simulink model "krause_model_bodine"  (R2017a)
settings: Solver=FixedStepAuto  StartTime=0.0  StopTime=0.4  FixedStep=1e-5  RelTol=1e-3
values from neighbouring files (symbols this model uses):
  B = 0.000124    [krause_model_params.m]
  J = 0.001    [krause_model_params.m]
  Llr = 0.0518    [krause_model_params.m]
  Lls = 0.0222    [krause_model_params.m]
  Lmlstar = 1/(1/Lls+1/Lm+1/Llr)    (= 0.0147655913289)    [krause_model_params.m]
  P = 4    [krause_model_params.m]
  Rr = 12.76    [krause_model_params.m]
  Rs = 14.6    [krause_model_params.m]
libraries: powerlib x12, simulink x1
settings Model: Creator=mircea  LastModifiedBy=mircea

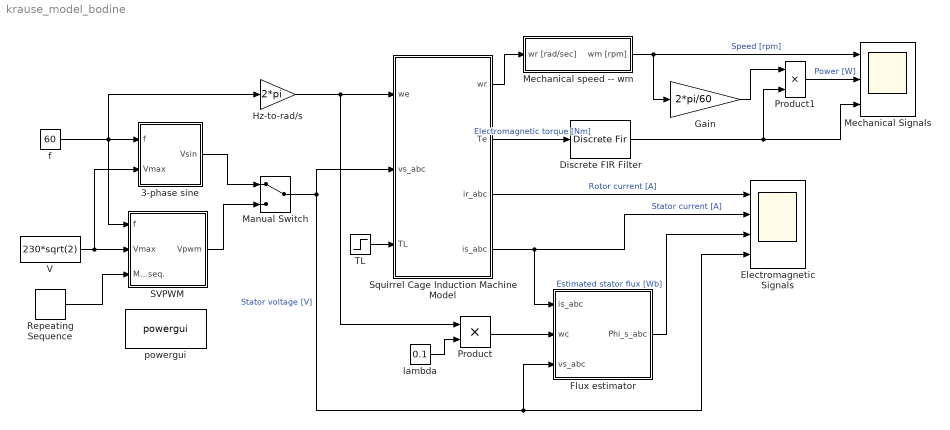
== system krause_model_bodine ==
  3-phase sine : Subsystem
  Discrete FIR Filter : DiscreteFir  Coefficients=ones(1,500)/500
  Electromagnetic Signals : Scope  NumInputPorts=4
  Flux estimator : Subsystem
  Gain : Gain  Gain=2*pi/60
  Hz-to-rad/s : Gain  Gain=2*pi
  Manual Switch : ManualSwitch
  Mechanical Signals : Scope  NumInputPorts=3
  "Mechanical speed -- wm" : Subsystem
  Product : Product
  Product1 : Product
  Repeating Sequence : simulink/Sources/Repeating Sequence  rep_seq_t=[0 0.25 0.5 0.75 1]/(10e3)  rep_seq_y=[1 0 -1 0 1]
  SVPWM : Subsystem
  Squirrel Cage Induction Machine Model : Subsystem
  TL : Step  Time=0.2  After=0.7602
  V : Constant  Value=230*sqrt(2)
  f : Constant  Value=60
  lambda : Constant  Value=0.1
  powergui : powerlib/powergui  Priority=1  SimulationMode=Discrete  SampleTime=1e-5  frequency=60  Iterations=50  frequencyindice=0  Pbase=100e6  ErrMax=1e-4  UnitsV=kV  UnitsW=MW  buscounter=0  FunctionMessages=off  echomessages=off  EnableUseOfTLC=off  CurrentSourceSwitches=off  DisableSnubberDevices=off  DisableRonSwitches=off  DisableVfSwitches=off  DisplayEquations=off  SolverType=Tustin/Backward Euler (TBE)  Interpol=off  ExternalGateDelay=off  methode=off  Ts=100  x0status=blocks  SPID=off  SwTol=0  HookPort=off  RestoreLinks=warning  ResistiveCurrentMeasurement=off  Frange=[0:2:500]  Ylog=off  Xlog=on  ShowGrid=off  save=off  variable=ZData  structure=0  ZoomFFT=off  StartTime=0.0  cycles=1  DisplayStyle=1  fundamental=60  FreqAxis=off  MaxFrequency=1000  frequencyindicesteady=1  RmsSteady=1  display=off
  wires:
  TL/1 -> Squirrel Cage Induction Machine Model/3(TL)
  Squirrel Cage Induction Machine Model/4(is_abc) -> Electromagnetic Signals/2, Flux estimator/1(is_abc)  "Stator current [A]"
  Squirrel Cage Induction Machine Model/3(ir_abc) -> Electromagnetic Signals/1  "Rotor current [A]"
  Product/1 -> Flux estimator/2(wc)
  Flux estimator/1(Phi_s_abc) -> Electromagnetic Signals/3  "Estimated stator flux [Wb]"
  f/1 -> 3-phase sine/1(f), SVPWM/1(f), Hz-to-rad/s/1
  lambda/1 -> Product/2
  Squirrel Cage Induction Machine Model/1(wr) -> "Mechanical speed -- wm"/1(wr [rad/sec])
  "Mechanical speed -- wm"/1(wm [rpm]) -> Mechanical Signals/1, Gain/1  "Speed [rpm]"
  V/1 -> 3-phase sine/2(Vmax), SVPWM/2(Vmax)
  Squirrel Cage Induction Machine Model/2(Te) -> Discrete FIR Filter/1  "Electromagnetic torque [Nm]"
  Product1/1 -> Mechanical Signals/2  "Power [W]"
  Gain/1 -> Product1/1
  Repeating Sequence/1 -> SVPWM/3(Mod. seq.)
  Hz-to-rad/s/1 -> Squirrel Cage Induction Machine Model/1(we), Product/1
  3-phase sine/1(Vsin) -> Manual Switch/1
  SVPWM/1(Vpwm) -> Manual Switch/2
  Manual Switch/1 -> Electromagnetic Signals/4, Flux estimator/3(vs_abc), Squirrel Cage Induction Machine Model/2(vs_abc)  "Stator voltage [V]"
  Discrete FIR Filter/1 -> Mechanical Signals/3, Product1/2

== system krause_model_bodine/3-phase sine ==
  f : Inport
  Vmax : Inport  Port=2
  Clock : Clock
  Constant4 : Constant  Value=2*pi/3*[ 0,-1,1 ]
  Hz-to-rad/s : Gain  Gain=2*pi  SaturateOnIntegerOverflow=on  OutDataTypeStr=Inherit: Same as input  ParamDataTypeStr=Inherit: Same as input
  Product : Product
  Product1 : Product  SaturateOnIntegerOverflow=on  InputSameDT=on  OutDataTypeStr=Inherit: Same as first input
  Sum1 : Sum  SaturateOnIntegerOverflow=on  InputSameDT=on  OutDataTypeStr=Inherit: Same as first input
  Trigonometric Function1 : Trigonometry
  Vsin : Outport
  wires:
  Constant4/1 -> Sum1/2
  Sum1/1 -> Trigonometric Function1/1
  Product1/1 -> Sum1/1
  Hz-to-rad/s/1 -> Product1/2
  Clock/1 -> Product1/1
  Trigonometric Function1/1 -> Product/2
  Vmax/1 -> Product/1
  Product/1 -> Vsin/1
  f/1 -> Hz-to-rad/s/1

== system krause_model_bodine/Flux estimator ==
  is_abc : Inport
  wc : Inport  Port=2
  vs_abc : Inport  Port=3
  Gain1 : Gain  Gain=Rs  SaturateOnIntegerOverflow=on  OutDataTypeStr=Inherit: Same as input  ParamDataTypeStr=Inherit: Same as input
  Integrator : Integrator
  Product : Product
  Subtract : Sum  Inputs=+-
  Sum : Sum  Inputs=|+-
  Phi_s_abc : Outport
  wires:
  Gain1/1 -> Subtract/2
  vs_abc/1 -> Subtract/1
  is_abc/1 -> Gain1/1
  Subtract/1 -> Sum/1
  Sum/1 -> Integrator/1
  Product/1 -> Sum/2
  wc/1 -> Product/2
  Integrator/1 -> Phi_s_abc/1, Product/1

== system krause_model_bodine/Mechanical speed -- wm ==
  wr [rad/sec] : Inport
  Gain : Gain  Gain=2/P
  Gain2 : Gain  Gain=30/pi
  wm [rpm] : Outport
  wires:
  Gain2/1 -> wm [rpm]/1  "wr rpm"
  wr [rad/sec]/1 -> Gain/1
  Gain/1 -> Gain2/1

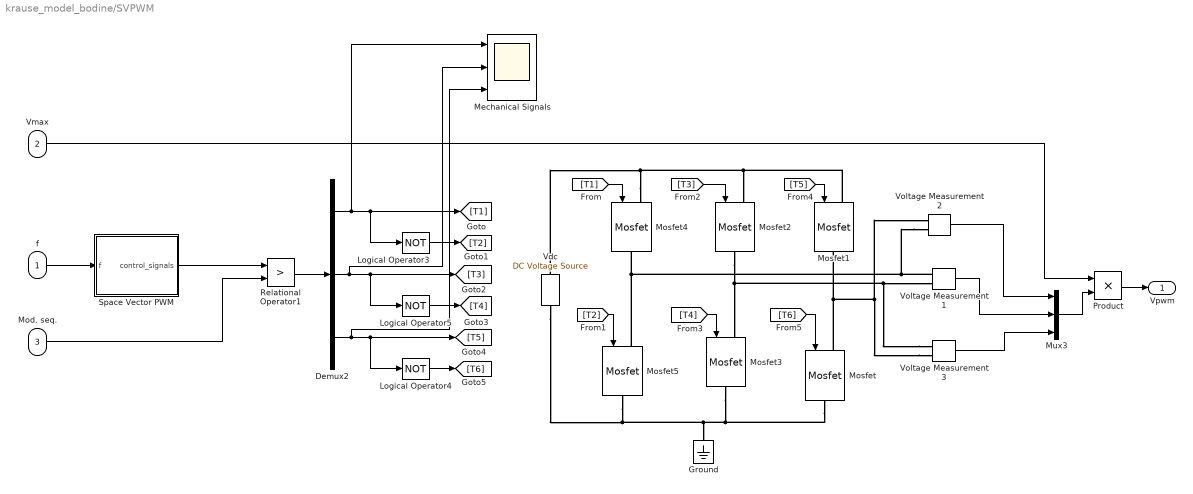
== system krause_model_bodine/SVPWM ==
  f : Inport
  Vmax : Inport  Port=2
  Mod. seq. : Inport  Port=3
  Demux2 : Demux  Outputs=3
  Ground : powerlib/Elements/Ground  LConnTagsString=a
  Logical Operator3 : Logic  Operator=NOT  AllPortsSameDT=off  OutDataTypeStr=boolean
  Logical Operator4 : Logic  Operator=NOT  AllPortsSameDT=off  OutDataTypeStr=boolean
  Logical Operator5 : Logic  Operator=NOT  AllPortsSameDT=off  OutDataTypeStr=boolean
  Mechanical Signals : Scope  NumInputPorts=3
  Mosfet{,1..5} (6 alike) : powerlib/Power Electronics/Mosfet  Ron=0.1  Lon=0  Rd=0.01  Vfd=0  IC=0  Rs=1e5  Cs=inf  Measurements=off
  Mux3 : Mux  Inputs=3
  Product : Product
  Relational Operator1 : RelationalOperator  Operator=>  RndMeth=Nearest
  Space Vector PWM : Subsystem
  Vdc : powerlib/Electrical Sources/DC Voltage Source  Amplitude=1  Measurements=None
  Voltage Measurement1 : powerlib/Measurements/Voltage Measurement  PhasorSimulation=off  OutputType=Complex  PSBequivalent=0
  Voltage Measurement2 : powerlib/Measurements/Voltage Measurement  PhasorSimulation=off  OutputType=Complex  PSBequivalent=0
  Voltage Measurement3 : powerlib/Measurements/Voltage Measurement  PhasorSimulation=off  OutputType=Complex  PSBequivalent=0
  Vpwm : Outport
  wires:
  [T6] -> Mosfet/1
  [T5] -> Mosfet1/1
  [T4] -> Mosfet3/1
  [T3] -> Mosfet2/1
  [T2] -> Mosfet5/1
  [T1] -> Mosfet4/1
  f/1 -> Space Vector PWM/1(f)
  Demux2/3 -> Mechanical Signals/3, [T5], Logical Operator4/1
  Demux2/2 -> Mechanical Signals/2, [T3], Logical Operator5/1
  Logical Operator5/1 -> [T4]
  Demux2/1 -> Mechanical Signals/1, [T1], Logical Operator3/1
  Space Vector PWM/1(control_signals) -> Relational Operator1/1
  Logical Operator4/1 -> [T6]
  Logical Operator3/1 -> [T2]
  Relational Operator1/1 -> Demux2/1
  Mod. seq./1 -> Relational Operator1/2
  Voltage Measurement2/1 -> Mux3/1
  Voltage Measurement1/1 -> Mux3/2
  Voltage Measurement3/1 -> Mux3/3
  Mux3/1 -> Product/2
  Vmax/1 -> Product/1
  Product/1 -> Vpwm/1
  connections:
  Voltage Measurement3/LConn2 -- Mosfet/LConn1 -- Mosfet1/RConn1 -- Voltage Measurement2/LConn1
  Mosfet4/LConn1 -- Mosfet1/LConn1 -- Mosfet2/LConn1 -- Vdc/RConn1
  Voltage Measurement3/LConn1 -- Mosfet3/LConn1 -- Mosfet2/RConn1 -- Voltage Measurement1/LConn2
  Mosfet5/RConn1 -- Mosfet/RConn1 -- Mosfet3/RConn1 -- Ground/LConn1 -- Vdc/LConn1
  Voltage Measurement2/LConn2 -- Voltage Measurement1/LConn1 -- Mosfet4/RConn1 -- Mosfet5/LConn1

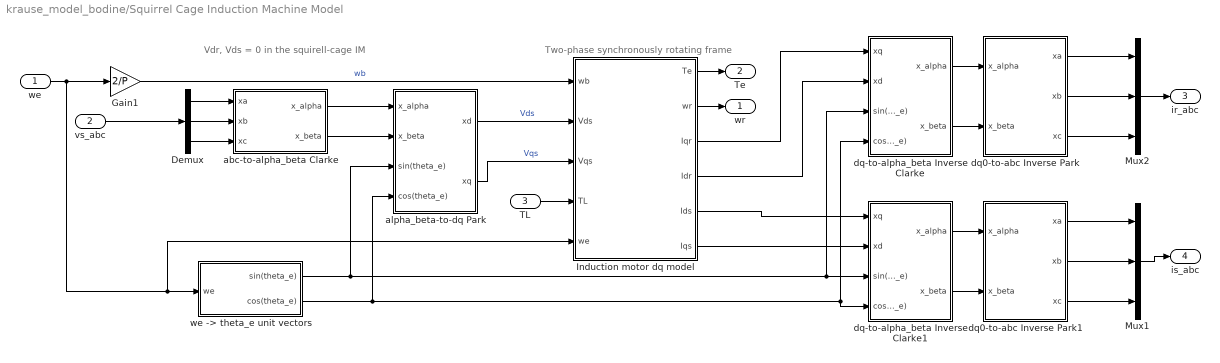
== system krause_model_bodine/Squirrel Cage Induction Machine Model ==
  note: Vdr, Vds = 0 in the squirell-cage IM
  note: Two-phase synchronously rotating frame
  we : Inport
  vs_abc : Inport  Port=2
  TL : Inport  Port=3
  Demux : Demux  Outputs=3
  Gain1 : Gain  Gain=2/P
  Induction motor dq model : Subsystem
  Mux1 : Mux  Inputs=3
  Mux2 : Mux  Inputs=3
  abc-to-alpha_beta Clarke : Subsystem
  alpha_beta-to-dq Park : Subsystem
  dq-to-alpha_beta Inverse Clarke : Subsystem
  dq-to-alpha_beta Inverse Clarke1 : Subsystem
  dq0-to-abc Inverse Park : Subsystem
  dq0-to-abc Inverse Park1 : Subsystem
  "we -> theta_e unit vectors" : Subsystem
  wr : Outport
  Te : Outport  Port=2
  ir_abc : Outport  Port=3
  is_abc : Outport  Port=4
  wires:
  Induction motor dq model/5(Ids) -> dq-to-alpha_beta Inverse Clarke1/1(xq)
  we/1 -> "we -> theta_e unit vectors"/1(we), Induction motor dq model/5(we), Gain1/1
  TL/1 -> Induction motor dq model/4(TL)
  alpha_beta-to-dq Park/2(xq) -> Induction motor dq model/3(Vqs)  "Vqs"
  "we -> theta_e unit vectors"/1(sin(theta_e)) -> dq-to-alpha_beta Inverse Clarke1/3(sin(theta_e)), dq-to-alpha_beta Inverse Clarke/3(sin(theta_e)), alpha_beta-to-dq Park/3(sin(theta_e))
  "we -> theta_e unit vectors"/2(cos(theta_e)) -> alpha_beta-to-dq Park/4(cos(theta_e)), dq-to-alpha_beta Inverse Clarke1/4(cos(theta_e)), dq-to-alpha_beta Inverse Clarke/4(cos(theta_e))
  alpha_beta-to-dq Park/1(xd) -> Induction motor dq model/2(Vds)  "Vds"
  Induction motor dq model/2(wr) -> wr/1
  Induction motor dq model/1(Te) -> Te/1
  vs_abc/1 -> Demux/1
  Demux/2 -> abc-to-alpha_beta Clarke/2(xb)
  Demux/1 -> abc-to-alpha_beta Clarke/1(xa)
  Demux/3 -> abc-to-alpha_beta Clarke/3(xc)
  Mux2/1 -> ir_abc/1
  dq0-to-abc Inverse Park/1(xa) -> Mux2/1
  dq0-to-abc Inverse Park/2(xb) -> Mux2/2
  dq0-to-abc Inverse Park/3(xc) -> Mux2/3
  Induction motor dq model/6(Iqs) -> dq-to-alpha_beta Inverse Clarke1/2(xd)
  Induction motor dq model/3(Iqr) -> dq-to-alpha_beta Inverse Clarke/1(xq)
  Induction motor dq model/4(Idr) -> dq-to-alpha_beta Inverse Clarke/2(xd)
  abc-to-alpha_beta Clarke/1(x_alpha) -> alpha_beta-to-dq Park/1(x_alpha)
  abc-to-alpha_beta Clarke/2(x_beta) -> alpha_beta-to-dq Park/2(x_beta)
  dq-to-alpha_beta Inverse Clarke/1(x_alpha) -> dq0-to-abc Inverse Park/1(x_alpha)
  dq-to-alpha_beta Inverse Clarke/2(x_beta) -> dq0-to-abc Inverse Park/2(x_beta)
  dq0-to-abc Inverse Park1/2(xb) -> Mux1/2
  dq0-to-abc Inverse Park1/1(xa) -> Mux1/1
  dq0-to-abc Inverse Park1/3(xc) -> Mux1/3
  Mux1/1 -> is_abc/1
  dq-to-alpha_beta Inverse Clarke1/2(x_beta) -> dq0-to-abc Inverse Park1/2(x_beta)
  dq-to-alpha_beta Inverse Clarke1/1(x_alpha) -> dq0-to-abc Inverse Park1/1(x_alpha)
  Gain1/1 -> Induction motor dq model/1(wb)  "wb"

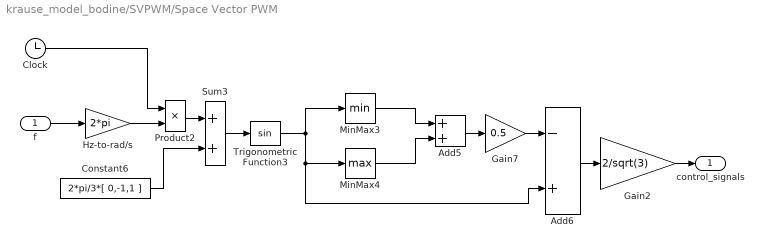
== system krause_model_bodine/SVPWM/Space Vector PWM ==
  f : Inport
  Add5 : Sum
  Add6 : Sum  Inputs=-+
  Clock : Clock
  Constant6 : Constant  Value=2*pi/3*[ 0,-1,1 ]
  Gain2 : Gain  Gain=2/sqrt(3)
  Gain7 : Gain  Gain=0.5
  Hz-to-rad/s : Gain  Gain=2*pi  SaturateOnIntegerOverflow=on  OutDataTypeStr=Inherit: Same as input  ParamDataTypeStr=Inherit: Same as input
  MinMax3 : MinMax
  MinMax4 : MinMax  Function=max
  Product2 : Product  SaturateOnIntegerOverflow=on  InputSameDT=on  OutDataTypeStr=Inherit: Same as first input
  Sum3 : Sum  SaturateOnIntegerOverflow=on  InputSameDT=on  OutDataTypeStr=Inherit: Same as first input
  Trigonometric Function3 : Trigonometry
  control_signals : Outport
  wires:
  Gain2/1 -> control_signals/1
  Trigonometric Function3/1 -> MinMax3/1, MinMax4/1, Add6/2
  Gain7/1 -> Add6/1
  f/1 -> Hz-to-rad/s/1
  Sum3/1 -> Trigonometric Function3/1
  Hz-to-rad/s/1 -> Product2/2
  MinMax3/1 -> Add5/1
  Constant6/1 -> Sum3/2
  Clock/1 -> Product2/1
  Add6/1 -> Gain2/1
  Add5/1 -> Gain7/1
  Product2/1 -> Sum3/1
  MinMax4/1 -> Add5/2

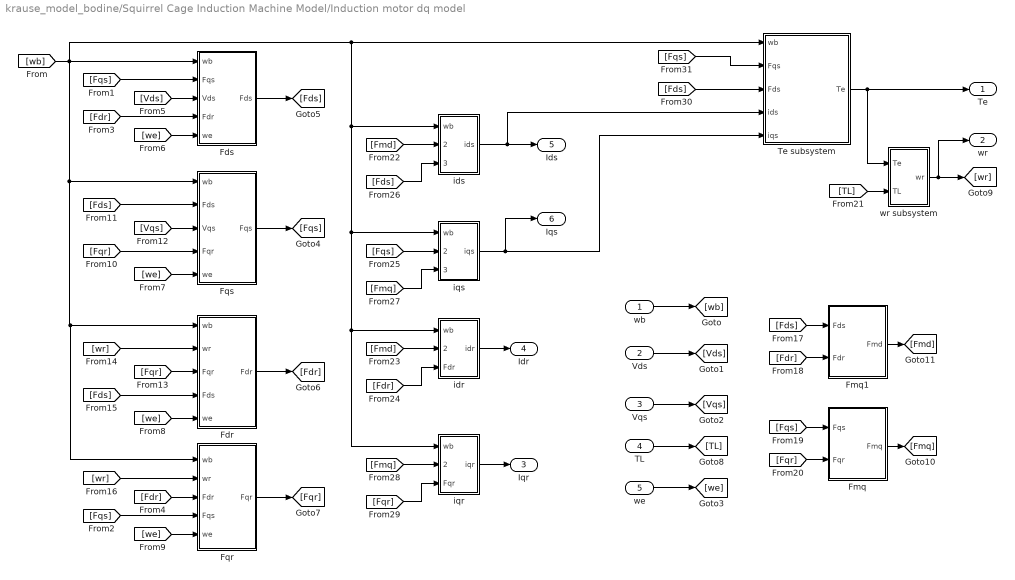
== system krause_model_bodine/Squirrel Cage Induction Machine Model/Induction motor dq model ==
  wb : Inport
  Vds : Inport  Port=2
  Vqs : Inport  Port=3
  TL : Inport  Port=4
  we : Inport  Port=5
  Fdr : Subsystem
  Fds : Subsystem
  Fmq : Subsystem
  Fmq1 : Subsystem
  Fqr : Subsystem
  Fqs : Subsystem
  Te subsystem : Subsystem
  idr : Subsystem
  ids : Subsystem
  iqr : Subsystem
  iqs : Subsystem
  wr subsystem : Subsystem
  Te : Outport
  wr : Outport  Port=2
  Iqr : Outport  Port=3
  Idr : Outport  Port=4
  Ids : Outport  Port=5
  Iqs : Outport  Port=6
  wires:
  Fmq1/1(Fmd) -> [Fmd]
  wb/1 -> [wb]
  Vds/1 -> [Vds]
  Vqs/1 -> [Vqs]
  we/1 -> [we]
  Fqs/1(Fqs) -> [Fqs]
  Fds/1(Fds) -> [Fds]
  Fdr/1(Fdr) -> [Fdr]
  Fqr/1(Fqr) -> [Fqr]
  [Fqs] -> Fds/2(Fqs)
  [Fqs] -> Fqr/4(Fqs)
  [Fdr] -> Fds/4(Fdr)
  [Vds] -> Fds/3(Vds)
  [we] -> Fds/5(we)
  [we] -> Fqs/5(we)
  [we] -> Fdr/5(we)
  [we] -> Fqr/5(we)
  [Fqr] -> Fqs/4(Fqr)
  [Fds] -> Fqs/2(Fds)
  [Vqs] -> Fqs/3(Vqs)
  [Fqr] -> Fdr/3(Fqr)
  [wr] -> Fdr/2(wr)
  [Fds] -> Fdr/4(Fds)
  [Fdr] -> Fqr/3(Fdr)
  [wr] -> Fqr/2(wr)
  [Fds] -> Fmq1/1(Fds)
  [Fdr] -> Fmq1/2(Fdr)
  [Fqs] -> Fmq/1(Fqs)
  [Fqr] -> Fmq/2(Fqr)
  TL/1 -> [TL]
  [TL] -> wr subsystem/2(TL)
  wr subsystem/1(wr) -> wr/1, [wr]
  [wb] -> Te subsystem/1(wb), iqs/1(wb), idr/1(wb), iqr/1(wb), ids/1(wb), Fqr/1(wb), Fdr/1(wb), Fqs/1(wb), Fds/1(wb)
  Fmq/1(Fmq) -> [Fmq]
  [Fmd] -> idr/2(Fmd)
  [Fqs] -> iqs/2(Fqs)
  [Fdr] -> idr/3(Fdr)
  [Fmd] -> ids/2(Fmd)
  [Fds] -> ids/3(Fds)
  [Fmq] -> iqs/3(Fmq)
  [Fmq] -> iqr/2(Fmq)
  [Fqr] -> iqr/3(Fqr)
  idr/1(idr) -> Idr/1
  iqr/1(iqr) -> Iqr/1
  ids/1(ids) -> Ids/1, Te subsystem/4(ids)
  iqs/1(iqs) -> Te subsystem/5(iqs), Iqs/1
  [Fds] -> Te subsystem/3(Fds)
  [Fqs] -> Te subsystem/2(Fqs)
  Te subsystem/1(Te) -> wr subsystem/1(Te), Te/1

== system krause_model_bodine/Squirrel Cage Induction Machine Model/abc-to-alpha_beta Clarke ==
  xa : Inport
  xb : Inport  Port=2
  xc : Inport  Port=3
  Demux2 : Demux  Outputs=2
  Gain1 : Gain  Gain=[1, 0, 0; 1/sqrt(3), 2/sqrt(3), 0]  Multiplication=Matrix(K*u) (u vector)
  Mux1 : Mux  Inputs=3
  x_alpha : Outport
  x_beta : Outport  Port=2
  wires:
  xa/1 -> Mux1/1
  xb/1 -> Mux1/2
  xc/1 -> Mux1/3
  Gain1/1 -> Demux2/1
  Mux1/1 -> Gain1/1
  Demux2/1 -> x_alpha/1  "x_alpha"
  Demux2/2 -> x_beta/1  "x_beta"

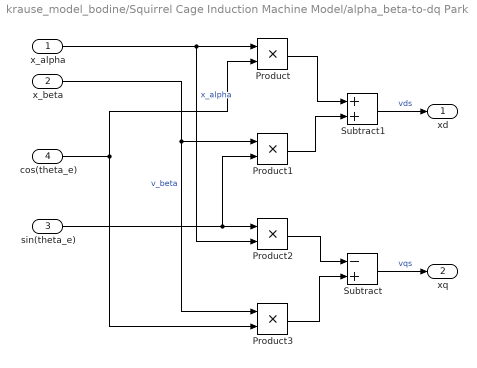
== system krause_model_bodine/Squirrel Cage Induction Machine Model/alpha_beta-to-dq Park ==
  x_alpha : Inport
  x_beta : Inport  Port=2
  sin(theta_e) : Inport  Port=3
  cos(theta_e) : Inport  Port=4
  Product{,1..3} (4 alike) : Product
  Subtract : Sum  Inputs=-+
  Subtract1 : Sum
  xd : Outport
  xq : Outport  Port=2
  wires:
  Subtract/1 -> xq/1  "vqs"
  Subtract1/1 -> xd/1  "vds"
  x_alpha/1 -> Product2/2, Product/1  "x_alpha"
  x_beta/1 -> Product3/1, Product1/1  "v_beta"
  cos(theta_e)/1 -> Product3/2, Product/2
  sin(theta_e)/1 -> Product2/1, Product1/2
  Product/1 -> Subtract1/1
  Product1/1 -> Subtract1/2
  Product2/1 -> Subtract/1
  Product3/1 -> Subtract/2

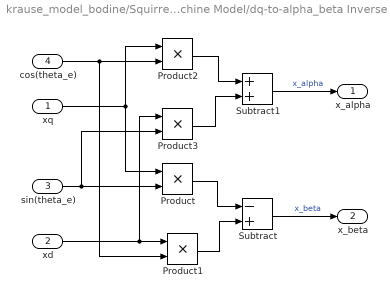
== system krause_model_bodine/Squirrel Cage Induction Machine Model/dq-to-alpha_beta Inverse Clarke ==
  xq : Inport
  xd : Inport  Port=2
  sin(theta_e) : Inport  Port=3
  cos(theta_e) : Inport  Port=4
  Product{,1..3} (4 alike) : Product
  Subtract : Sum  Inputs=-+
  Subtract1 : Sum
  x_alpha : Outport
  x_beta : Outport  Port=2
  wires:
  xd/1 -> Product3/1, Product1/1
  Product/1 -> Subtract/1
  Product1/1 -> Subtract/2
  Product2/1 -> Subtract1/1
  Product3/1 -> Subtract1/2
  xq/1 -> Product/1, Product2/1
  cos(theta_e)/1 -> Product2/2, Product1/2
  sin(theta_e)/1 -> Product3/2, Product/2
  Subtract1/1 -> x_alpha/1  "x_alpha"
  Subtract/1 -> x_beta/1  "x_beta"

== system krause_model_bodine/Squirrel Cage Induction Machine Model/dq-to-alpha_beta Inverse Clarke1 ==
  xq : Inport
  xd : Inport  Port=2
  sin(theta_e) : Inport  Port=3
  cos(theta_e) : Inport  Port=4
  Product{,1..3} (4 alike) : Product
  Subtract : Sum  Inputs=-+
  Subtract1 : Sum
  x_alpha : Outport
  x_beta : Outport  Port=2
  wires:
  xd/1 -> Product3/1, Product1/1
  Product/1 -> Subtract/1
  Product1/1 -> Subtract/2
  Product2/1 -> Subtract1/1
  Product3/1 -> Subtract1/2
  xq/1 -> Product/1, Product2/1
  cos(theta_e)/1 -> Product2/2, Product1/2
  sin(theta_e)/1 -> Product3/2, Product/2
  Subtract1/1 -> x_alpha/1  "x_alpha"
  Subtract/1 -> x_beta/1  "x_beta"

== system krause_model_bodine/Squirrel Cage Induction Machine Model/dq0-to-abc Inverse Park ==
  x_alpha : Inport
  x_beta : Inport  Port=2
  Demux2 : Demux  Outputs=3
  Gain1 : Gain  Gain=[1, 0; -1/2, sqrt(3)/2; -1/2, -sqrt(3)/2]  Multiplication=Matrix(K*u) (u vector)
  Mux1 : Mux  Inputs=2
  xa : Outport
  xb : Outport  Port=2
  xc : Outport  Port=3
  wires:
  Gain1/1 -> Demux2/1
  Demux2/1 -> xa/1
  x_alpha/1 -> Mux1/1
  x_beta/1 -> Mux1/2
  Mux1/1 -> Gain1/1
  Demux2/3 -> xb/1
  Demux2/2 -> xc/1

== system krause_model_bodine/Squirrel Cage Induction Machine Model/dq0-to-abc Inverse Park1 ==
  x_alpha : Inport
  x_beta : Inport  Port=2
  Demux2 : Demux  Outputs=3
  Gain1 : Gain  Gain=[1, 0; -1/2, sqrt(3)/2; -1/2, -sqrt(3)/2]  Multiplication=Matrix(K*u) (u vector)
  Mux1 : Mux  Inputs=2
  xa : Outport
  xb : Outport  Port=2
  xc : Outport  Port=3
  wires:
  Gain1/1 -> Demux2/1
  Demux2/1 -> xa/1
  x_alpha/1 -> Mux1/1
  x_beta/1 -> Mux1/2
  Mux1/1 -> Gain1/1
  Demux2/3 -> xb/1
  Demux2/2 -> xc/1

== system krause_model_bodine/Squirrel Cage Induction Machine Model/we -> theta_e unit vectors ==
  we : Inport
  Integrator : Integrator
  cos : Trigonometry  Operator=cos
  sin : Trigonometry
  sin(theta_e) : Outport
  cos(theta_e) : Outport  Port=2
  wires:
  sin/1 -> sin(theta_e)/1
  we/1 -> Integrator/1
  Integrator/1 -> sin/1, cos/1
  cos/1 -> cos(theta_e)/1

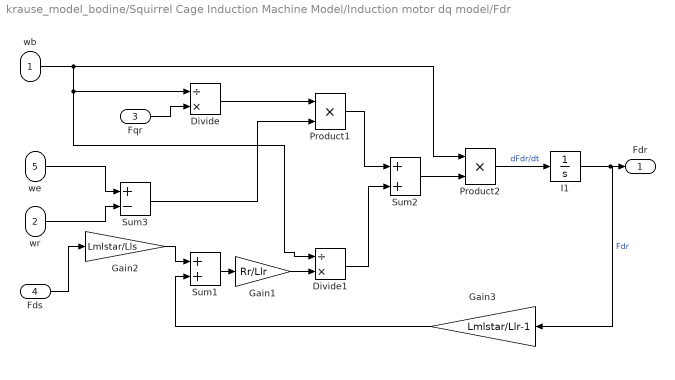
== system krause_model_bodine/Squirrel Cage Induction Machine Model/Induction motor dq model/Fdr ==
  wb : Inport
  wr : Inport  Port=2
  Fqr : Inport  Port=3
  Fds : Inport  Port=4
  we : Inport  Port=5
  Divide : Product  Inputs=/*
  Divide1 : Product  Inputs=/*
  Gain1 : Gain  Gain=Rr/Llr
  Gain2 : Gain  Gain=Lmlstar/Lls
  Gain3 : Gain  Gain=Lmlstar/Llr-1
  I1 : Integrator
  Product1 : Product
  Product2 : Product
  Sum1 : Sum
  Sum2 : Sum
  Sum3 : Sum  Inputs=+-
  Fdr : Outport
  wires:
  Sum2/1 -> Product2/2
  Product2/1 -> I1/1  "dFdr/dt"
  I1/1 -> Gain3/1, Fdr/1  "Fdr"
  wb/1 -> Divide1/1, Divide/1, Product2/1
  Fqr/1 -> Divide/2
  Sum1/1 -> Gain1/1
  Fds/1 -> Gain2/1
  Gain2/1 -> Sum1/1
  Gain3/1 -> Sum1/2
  we/1 -> Sum3/1
  wr/1 -> Sum3/2
  Divide/1 -> Product1/1
  Sum3/1 -> Product1/2
  Product1/1 -> Sum2/1
  Gain1/1 -> Divide1/2
  Divide1/1 -> Sum2/2

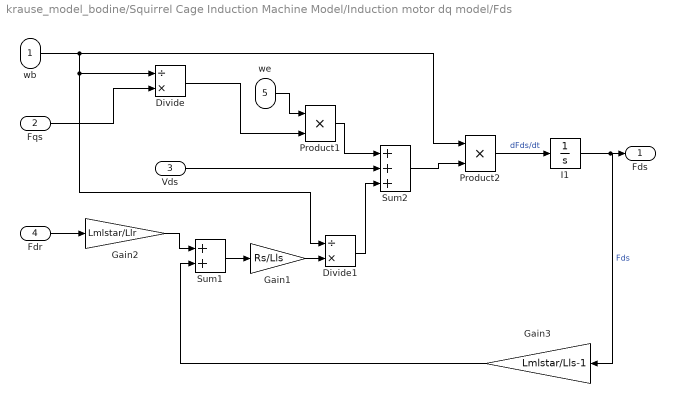
== system krause_model_bodine/Squirrel Cage Induction Machine Model/Induction motor dq model/Fds ==
  wb : Inport
  Fqs : Inport  Port=2
  Vds : Inport  Port=3
  Fdr : Inport  Port=4
  we : Inport  Port=5
  Divide : Product  Inputs=/*
  Divide1 : Product  Inputs=/*
  Gain1 : Gain  Gain=Rs/Lls
  Gain2 : Gain  Gain=Lmlstar/Llr
  Gain3 : Gain  Gain=Lmlstar/Lls-1
  I1 : Integrator
  Product1 : Product
  Product2 : Product
  Sum1 : Sum
  Sum2 : Sum  Inputs=+++
  Fds : Outport
  wires:
  Sum2/1 -> Product2/2
  Vds/1 -> Sum2/2
  Product2/1 -> I1/1  "dFds/dt"
  I1/1 -> Gain3/1, Fds/1  "Fds"
  wb/1 -> Product2/1, Divide1/1, Divide/1
  Fqs/1 -> Divide/2
  Divide/1 -> Product1/2
  Sum1/1 -> Gain1/1
  Fdr/1 -> Gain2/1
  Gain2/1 -> Sum1/1
  Gain3/1 -> Sum1/2
  we/1 -> Product1/1
  Product1/1 -> Sum2/1
  Gain1/1 -> Divide1/2
  Divide1/1 -> Sum2/3

== system krause_model_bodine/Squirrel Cage Induction Machine Model/Induction motor dq model/Fmq ==
  Fqs : Inport
  Fqr : Inport  Port=2
  Gain1 : Gain  Gain=1/Lls
  Gain2 : Gain  Gain=1/Llr
  Gain3 : Gain  Gain=Lmlstar
  Sum1 : Sum
  Fmq : Outport
  wires:
  Fqr/1 -> Gain2/1
  Fqs/1 -> Gain1/1
  Gain2/1 -> Sum1/2
  Gain1/1 -> Sum1/1
  Sum1/1 -> Gain3/1
  Gain3/1 -> Fmq/1

== system krause_model_bodine/Squirrel Cage Induction Machine Model/Induction motor dq model/Fmq1 ==
  Fds : Inport
  Fdr : Inport  Port=2
  Gain1 : Gain  Gain=1/Lls
  Gain2 : Gain  Gain=1/Llr
  Gain3 : Gain  Gain=Lmlstar
  Sum1 : Sum
  Fmd : Outport
  wires:
  Fdr/1 -> Gain2/1
  Fds/1 -> Gain1/1
  Gain2/1 -> Sum1/2
  Gain1/1 -> Sum1/1
  Sum1/1 -> Gain3/1
  Gain3/1 -> Fmd/1

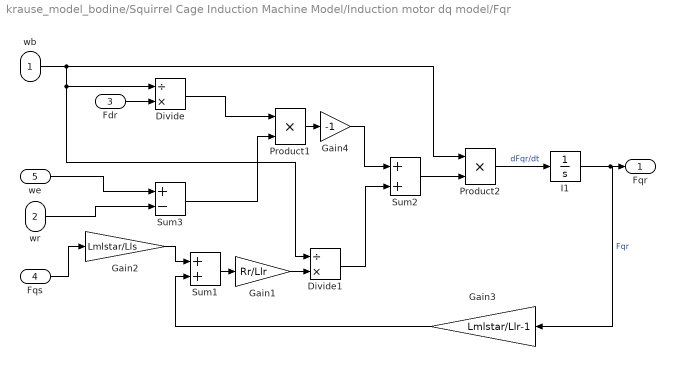
== system krause_model_bodine/Squirrel Cage Induction Machine Model/Induction motor dq model/Fqr ==
  wb : Inport
  wr : Inport  Port=2
  Fdr : Inport  Port=3
  Fqs : Inport  Port=4
  we : Inport  Port=5
  Divide : Product  Inputs=/*
  Divide1 : Product  Inputs=/*
  Gain1 : Gain  Gain=Rr/Llr
  Gain2 : Gain  Gain=Lmlstar/Lls
  Gain3 : Gain  Gain=Lmlstar/Llr-1
  Gain4 : Gain  Gain=-1
  I1 : Integrator
  Product1 : Product
  Product2 : Product
  Sum1 : Sum
  Sum2 : Sum
  Sum3 : Sum  Inputs=+-
  Fqr : Outport
  wires:
  Sum2/1 -> Product2/2
  Product2/1 -> I1/1  "dFqr/dt"
  I1/1 -> Gain3/1, Fqr/1  "Fqr"
  wb/1 -> Product2/1, Divide/1, Divide1/1
  Fdr/1 -> Divide/2
  Sum1/1 -> Gain1/1
  Fqs/1 -> Gain2/1
  Gain2/1 -> Sum1/1
  Gain3/1 -> Sum1/2
  we/1 -> Sum3/1
  wr/1 -> Sum3/2
  Divide/1 -> Product1/1
  Sum3/1 -> Product1/2
  Product1/1 -> Gain4/1
  Gain4/1 -> Sum2/1
  Gain1/1 -> Divide1/2
  Divide1/1 -> Sum2/2

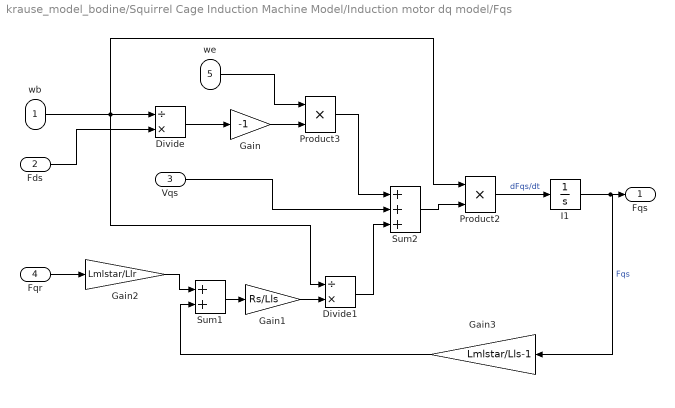
== system krause_model_bodine/Squirrel Cage Induction Machine Model/Induction motor dq model/Fqs ==
  wb : Inport
  Fds : Inport  Port=2
  Vqs : Inport  Port=3
  Fqr : Inport  Port=4
  we : Inport  Port=5
  Divide : Product  Inputs=/*
  Divide1 : Product  Inputs=/*
  Gain : Gain  Gain=-1
  Gain1 : Gain  Gain=Rs/Lls
  Gain2 : Gain  Gain=Lmlstar/Llr
  Gain3 : Gain  Gain=Lmlstar/Lls-1
  I1 : Integrator
  Product2 : Product
  Product3 : Product
  Sum1 : Sum
  Sum2 : Sum  Inputs=+++
  Fqs : Outport
  wires:
  Sum2/1 -> Product2/2
  Vqs/1 -> Sum2/2
  Product2/1 -> I1/1  "dFqs/dt"
  I1/1 -> Gain3/1, Fqs/1  "Fqs"
  wb/1 -> Divide/1, Divide1/1, Product2/1
  Fds/1 -> Divide/2
  Divide/1 -> Gain/1
  Sum1/1 -> Gain1/1
  Fqr/1 -> Gain2/1
  Gain2/1 -> Sum1/1
  Gain3/1 -> Sum1/2
  we/1 -> Product3/1
  Gain/1 -> Product3/2
  Product3/1 -> Sum2/1
  Gain1/1 -> Divide1/2
  Divide1/1 -> Sum2/3

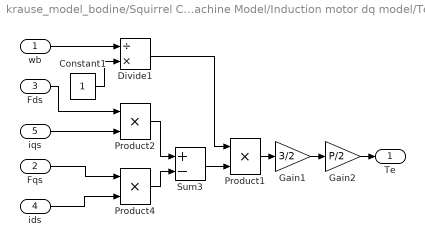
== system krause_model_bodine/Squirrel Cage Induction Machine Model/Induction motor dq model/Te subsystem ==
  wb : Inport
  Fqs : Inport  Port=2
  Fds : Inport  Port=3
  ids : Inport  Port=4
  iqs : Inport  Port=5
  Constant1 : Constant
  Divide1 : Product  Inputs=/*
  Gain1 : Gain  Gain=3/2
  Gain2 : Gain  Gain=P/2
  Product1 : Product
  Product2 : Product
  Product4 : Product
  Sum3 : Sum  Inputs=+-
  Te : Outport
  wires:
  Fds/1 -> Product2/1
  iqs/1 -> Product2/2
  wb/1 -> Divide1/1
  Fqs/1 -> Product4/1
  ids/1 -> Product4/2
  Product2/1 -> Sum3/1
  Product4/1 -> Sum3/2
  Sum3/1 -> Product1/2
  Gain1/1 -> Gain2/1
  Divide1/1 -> Product1/1
  Product1/1 -> Gain1/1
  Gain2/1 -> Te/1
  Constant1/1 -> Divide1/2

== system krause_model_bodine/Squirrel Cage Induction Machine Model/Induction motor dq model/idr ==
  wb : Inport
  Fmd : Inport  Port=2
  Fdr : Inport  Port=3
  Divide1 : Product  Inputs=/*
  Gain : Gain  Gain=1/Llr
  Sum1 : Sum  Inputs=+-
  idr : Outport
  wires:
  Sum1/1 -> Gain/1
  Fmd/1 -> Sum1/2
  Fdr/1 -> Sum1/1
  Gain/1 -> Divide1/2
  Divide1/1 -> idr/1
  wb/1 -> Divide1/1

== system krause_model_bodine/Squirrel Cage Induction Machine Model/Induction motor dq model/ids ==
  wb : Inport
  Fmd : Inport  Port=2
  Fds : Inport  Port=3
  Divide1 : Product  Inputs=/*
  Gain : Gain  Gain=1/Lls
  Sum1 : Sum  Inputs=+-
  ids : Outport
  wires:
  Sum1/1 -> Gain/1
  Fmd/1 -> Sum1/2
  Fds/1 -> Sum1/1
  Gain/1 -> Divide1/2
  Divide1/1 -> ids/1
  wb/1 -> Divide1/1

== system krause_model_bodine/Squirrel Cage Induction Machine Model/Induction motor dq model/iqr ==
  wb : Inport
  Fmq : Inport  Port=2
  Fqr : Inport  Port=3
  Divide1 : Product  Inputs=/*
  Gain : Gain  Gain=1/Llr
  Sum1 : Sum  Inputs=+-
  iqr : Outport
  wires:
  Sum1/1 -> Gain/1
  Fmq/1 -> Sum1/2
  Fqr/1 -> Sum1/1
  Divide1/1 -> iqr/1
  Gain/1 -> Divide1/2
  wb/1 -> Divide1/1

== system krause_model_bodine/Squirrel Cage Induction Machine Model/Induction motor dq model/iqs ==
  wb : Inport
  Fqs : Inport  Port=2
  Fmq : Inport  Port=3
  Divide1 : Product  Inputs=/*
  Gain : Gain  Gain=1/Lls
  Sum1 : Sum  Inputs=+-
  iqs : Outport
  wires:
  Sum1/1 -> Gain/1
  Fmq/1 -> Sum1/2
  Fqs/1 -> Sum1/1
  Gain/1 -> Divide1/2
  Divide1/1 -> iqs/1
  wb/1 -> Divide1/1

== system krause_model_bodine/Squirrel Cage Induction Machine Model/Induction motor dq model/wr subsystem ==
  note: Mechanical speed model with friction
  Te : Inport
  TL : Inport  Port=2
  Gain : Gain  Gain=P/2
  Gain1 : Gain  Gain=B
  Gain2 : Gain  Gain=1/J
  Integrator : Integrator
  Sum1 : Sum  Inputs=+-
  Sum2 : Sum  Inputs=+-
  wr : Outport
  wires:
  Sum1/1 -> Gain/1
  TL/1 -> Sum1/2
  Te/1 -> Sum1/1
  Gain1/1 -> Sum2/2
  Gain/1 -> Sum2/1
  Integrator/1 -> Gain1/1, wr/1
  Sum2/1 -> Gain2/1
  Gain2/1 -> Integrator/1
